simulink model "ClosedLoopPMSM_ASMO_MPC"  (R2023b)
settings: Solver=ode4  StartTime=0.0  StopTime=3  FixedStep=1e-6  RelTol=1e-4
InitFcn:
  | Vdc=24;
  | Rs=0.05734;
  | Ld=1.8166e-05;
  | Lq=1.8166e-05;
  | Ls=1.8166e-05;
  | pm=0.0185;
  | P=14;
  | B=1e-4;
  | J=2.94e-5;
  | Tpwm=30e-6;
  | 
  | fc=20;
  | mag_vel=100;
undefined symbols (not defined in the file): DiscIntNeverNeededParam
libraries: simulink x3, spsThreePhaseVIMeasurementLib x2, spsDCVoltageSourceLib x2, slpidlib x2, spsThreeLevelBridgeLib x1, spsUniversalBridgeLib x1, spsPermanentMagnetSynchronousMachineLib x1, sps_lib x1
(part 1 of 2)
settings Model: Creator=Admin  LastModifiedBy=Admin
settings SolverCC: AlgebraicLoopSolver=TrustRegion
settings DataIOCC: ReturnWorkspaceOutputs=off
settings OptimizationCC: LifeSpan=inf
settings DebuggingCC: UnconnectedInputMsg=warning  UnconnectedOutputMsg=warning  UnconnectedLineMsg=warning  SFUnexpectedBacktrackingDiag=warning  SFNoUnconditionalDefaultTransitionDiag=warning  ArithmeticOperatorsInVariantConditions=warning
settings ModelReferenceCC: EnableRefExpFcnMdlSchedulingChecks=on
settings SFSimCC: SimUseLocalCustomCode=off  CustomCodeUndefinedFunction=UseInterfaceOnly
settings RTWCC: RTWUseLocalCustomCode=off
settings CodeAppCC: StateflowObjectComments=on
settings GRTTargetCC: TargetLangStandard=C89/C90 (ANSI)
settings ConfigComp: CovMetricSettings=dw  CovSaveCumulativeToWorkspaceVar=on  CovSaveSingleToWorkspaceVar=on  CovExternalEMLEnable=off
settings SimscapeCC: SimscapeNormalizeSystem=off

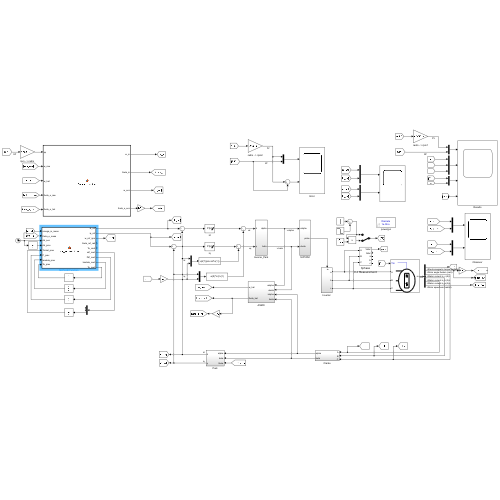
[thumbnail: Simulink's stored preview of the top-level diagram]
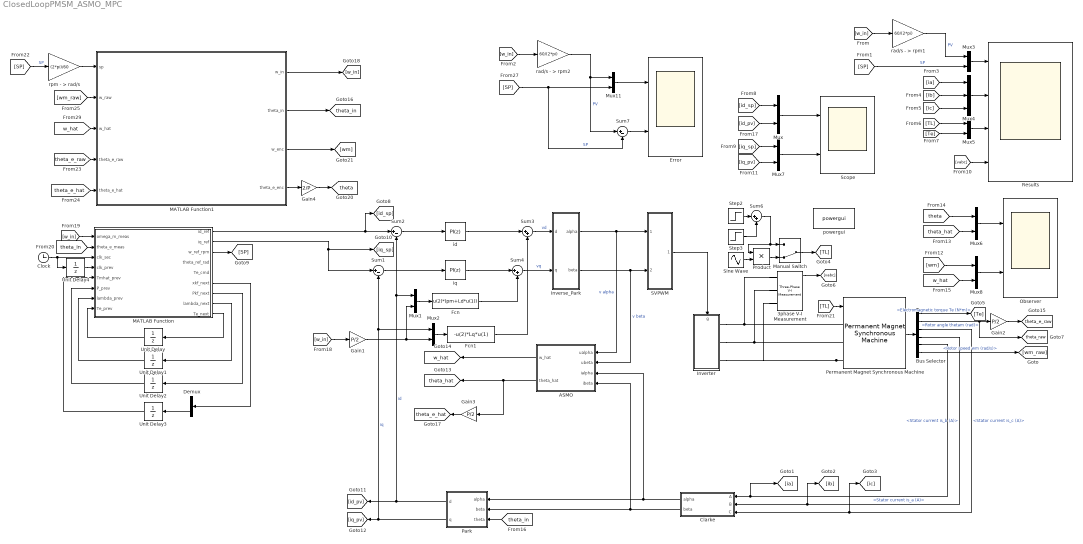
== system ClosedLoopPMSM_ASMO_MPC ==
  3phase V-I Measurement : spsThreePhaseVIMeasurementLib/Three-Phase V-I Measurement  VoltageMeasurement=phase-to-phase  SetLabelV=off  LabelV=Vabc  Vpu=off  VpuLL=off  CurrentMeasurement=yes  SetLabelI=off  LabelI=Iabc  Ipu=off  Pbase=100e6  Vbase=500e3  OutputType=Complex  PhasorSimulation=off  PSBequivalent=0
  ASMO : Subsystem
  Bus Selector : BusSelector  OutputSignals=Electromagnetic torque Te (N*m),Rotor angle thetam (rad),Stator current is_c (A),Stator current is_b (A),Stator current is_a (A),Rotor speed wm (rad/s)
  Clarke : Subsystem
  Clock : Clock
      settings: Decimation=33
  Demux : Demux  Outputs=3
  Error : Scope  NumInputPorts=2
  Fcn : Fcn  Expr=u(2)*(pm+Ld*u(1))
  Fcn1 : Fcn  Expr=-u(2)*Lq*u(1)
  Gain1 : Gain  Gain=P/2
  Gain2 : Gain  Gain=P/2
  Gain3 : Gain  Gain=P/2
  Gain4 : Gain  Gain=2/P
  Inverse_Park : Subsystem
  Inverter : Subsystem
      settings: PortSchema="{\"entries\":[{\"content\":{\"sides\":[{\"content\":{},\"type\":\"ConnectorPlacement.EquallySpacedRectSide\",\"uuid\":\"187c6bc1-a8de-4289-8015-4317398378bc\"},{\"content\":{\"connectorIds\":[\"RConn1\",\"RConn2\",\"RConn3\"],\"side\":\"RIGHT\"},\"type\":\"ConnectorPlacement.EquallySpacedRectSide\",\"uuid\":\"9f177a2c-a1b4-485f-9b91-a35efcc62074\"},{\"content\":{\"connectorIds\":[\"In1\"],\"side\":\"TOP\"},\"type\":\"ConnectorPlacement.EquallySpacedRectSide\",\"uuid\":\"7cd38b0a-0afe-4879-8b43-8c0c1c17e55c\"}]},\"type\":\"ConnectorPlacement.EquallySpacedConnector\",\"uuid\":\"53672e9b-5b63-4df3-a21b-cd886d268e09\"}],\"packageUris\":[\"http://schema.mathworks.com/mf0/Connector/R2020b\"],\"version\":\"1.0\"}"
  MATLAB Function : MATLAB Function  TreatAsAtomicUnit=on
  MATLAB Function1 : MATLAB Function  TreatAsAtomicUnit=on
  Manual Switch : ManualSwitch  CurrentSetting=0
  Mux{,1..3,5..8,11} (9 alike) : Mux  Inputs=2
  Mux4 : Mux  Inputs=3
  Observer : Scope  NumInputPorts=2
  Park : Subsystem
  Permanent Magnet Synchronous Machine : spsPermanentMagnetSynchronousMachineLib/Permanent Magnet Synchronous Machine  NbPhases=3  FluxDistribution=Sinusoidal  RotorType=Salient-pole  MechanicalLoad=Torque Tm  PresetModel=No  ShowDetailedParameters=on  MeasurementBus=off  Resistance=Rs  Inductance=8.5e-3  dqInductances=[Ld,Lq]  La=0.000395  MachineConstant=Flux linkage established by magnets (V.s)  Flux=pm  VoltageCst=23.4887  TorqueCst=0.19425  Flat=120  Mechanical=[J B P/2]  PolePairs=4  InitialConditions=[0,0, 0,0]  InitialConditions5ph=[0 0 0 0 0 0]  RefAngle=Aligned with phase A axis (original Park)  IterativeDiscreteModel=Trapezoidal non iterative  TsBlock=-1  TsPowergui=0
  Product : Product
  Results : Scope  NumInputPorts=4
  SVPWM : Subsystem
  Scope : Scope  NumInputPorts=2
  Sine Wave : Sin  Frequency=62.83  SampleTime=0
  Step2 : Step  Time=0.1  After=0.1  SampleTime=0
  Step3 : Step  Time=0.15  After=-0.1  SampleTime=0
  Sum1 : Sum  Inputs=|+-
  Sum2 : Sum  Inputs=|+-
  Sum3 : Sum  Inputs=|++
  Sum4 : Sum  Inputs=|++
  Sum6 : Sum  Inputs=|++
  Sum7 : Sum  Inputs=|+-
  Unit Delay : UnitDelay  SampleTime=30e-6  HasFrameUpgradeWarning=on
  Unit Delay1 : UnitDelay  InitialCondition=zeros(16,1)  SampleTime=30e-6  HasFrameUpgradeWarning=on
  Unit Delay2 : UnitDelay  InitialCondition=reshape([1 0 0; 0 1 0; 0 0 1], 9, 1)  SampleTime=30e-6  HasFrameUpgradeWarning=on
  Unit Delay3 : UnitDelay  SampleTime=30e-6  HasFrameUpgradeWarning=on
  Unit Delay4 : UnitDelay  SampleTime=30e-6  HasFrameUpgradeWarning=on
  id : slpidlib/PID Controller  Controller=PI  Form=Parallel  TimeDomain=Discrete-time  UseExternalTs=off  SampleTime=-1  IntegratorMethod=Forward Euler  FilterMethod=Forward Euler  ControllerParametersSource=internal  P=0.02283e4  I=72.06e1  UseKiTs=off  D=0  N=100  UseFilter=on  TunerSelectOption=Transfer Function Based (PID Tuner App)  InitialConditionSource=internal  InitialConditionForIntegrator=0  InitialConditionForFilter=0  DifferentiatorICPrevScaledInput=0  ExternalReset=none  TrackingMode=off  Kt=1  LimitOutput=on  SatLimitsSource=internal  UpperSaturationLimit=30  LowerSaturationLimit=-30  LinearizeAsGain=off  AntiWindupMode=clamping  Kb=1  LimitIntegrator=off  UpperIntegratorSaturationLimit=inf  LowerIntegratorSaturationLimit=-inf  POutMin=[]  POutMax=[]  IOutMin=[]  IOutMax=[]  DOutMin=[]  DOutMax=[]  NOutMin=[]  NOutMax=[]  SumOutMin=[]  SumOutMax=[]  SaturationOutMin=[]  SaturationOutMax=[]  PParamMin=[]  PParamMax=[]  IParamMin=[]  IParamMax=[]  DParamMin=[]  DParamMax=[]  NParamMin=[]  NParamMax=[]  KbParamMin=[]  KbParamMax=[]  KtParamMin=[]  KtParamMax=[]  KbOutMin=[]  KbOutMax=[]  KtOutMin=[]  KtOutMax=[]  IntegratorOutMin=[]  IntegratorOutMax=[]  FilterOutMin=[]  FilterOutMax=[]  SumI1OutMin=[]  SumI1OutMax=[]  SumI2OutMin=[]  SumI2OutMax=[]  SumI3OutMin=[]  SumI3OutMax=[]  SumI4OutMin=[]  SumI4OutMax=[]  SumDOutMin=[]  SumDOutMax=[]  DifferentiatorOutMin=[]  DifferentiatorOutMax=[]  FilterDiffOutCoefMin=[]  FilterDiffOutCoefMax=[]  ReciprocalOutMin=[]  ReciprocalOutMax=[]  SumDenOutMin=[]  SumDenOutMax=[]  SumNumOutMin=[]  SumNumOutMax=[]  DivideOutMin=[]  DivideOutMax=[]  UdiffTsProdOutMin=[]  UdiffTsProdOutMax=[]  NTsProdOutMin=[]  NTsProdOutMax=[]  UintegralTsProdOutMin=[]  UintegralTsProdOutMax=[]  UngainTsProdOutMin=[]  UngainTsProdOutMax=[]  ClampingZeroOutDataTypeStr=Inherit: Inherit via back propagation  ClampingZeroOutMin=[]  ClampingZeroOutMax=[]  FilterDenConstantOutDataTypeStr=Inherit: Inherit via back propagation  FilterDenConstantOutMin=[]  FilterDenConstantOutMax=[]  PCopyOutDataTypeStr=Inherit: Inherit via back propagation  PCopyOutMin=[]  PCopyOutMax=[]  NCopyOutDataTypeStr=Inherit: Inherit via back propagation  NCopyOutMin=[]  NCopyOutMax=[]  IntegratorContinuousStateAttributes=''  IntegratorStateMustResolveToSignalObject=off  IntegratorRTWStateStorageClass=Auto  FilterContinuousStateAttributes=''  FilterStateMustResolveToSignalObject=off  FilterRTWStateStorageClass=Auto  ParallelPVariant=InternalParameters  IdealPVariant=Disabled  IVariant=InternalParameters  DVariant=Disabled  IntegratorVariant=Discrete  SatVariant=Enabled  AWVariant=DiscClampingParallel  PCopyVariant=Disabled  TRVariant=Disabled  FdbkBlocksVariant=Forward  IdealPFdbkVariant=Disabled  SatFdbkVariant=Disabled  DerivativeFilterVariant=Disabled  NVariant=Disabled  NCopyVariant=Disabled_SignalSpec  FilterICVariant=Disabled  IntegratorICVariant=InternalICs  ExternalResetVariant=Disabled  TRSumVariant=Passthrough  SumFdbkVariant=Disabled  SumVariant=Sum_PI  TsampFilterVariant=InternalTs  TsampNgainVariant=Passthrough  TsampIntegralVariant=Disabled_SignalSpec  ExternalSaturationOutDataTypeStr=Inherit: Same as second input
  iq : slpidlib/PID Controller  Controller=PI  Form=Parallel  TimeDomain=Discrete-time  UseExternalTs=off  SampleTime=-1  IntegratorMethod=Forward Euler  FilterMethod=Forward Euler  ControllerParametersSource=internal  P=0.02283e4  I=72.06e1  UseKiTs=off  D=0  N=100  UseFilter=on  TunerSelectOption=Transfer Function Based (PID Tuner App)  InitialConditionSource=internal  InitialConditionForIntegrator=0  InitialConditionForFilter=0  DifferentiatorICPrevScaledInput=0  ExternalReset=none  TrackingMode=off  Kt=1  LimitOutput=on  SatLimitsSource=internal  UpperSaturationLimit=30  LowerSaturationLimit=-30  LinearizeAsGain=off  AntiWindupMode=clamping  Kb=1  LimitIntegrator=off  UpperIntegratorSaturationLimit=inf  LowerIntegratorSaturationLimit=-inf  POutMin=[]  POutMax=[]  IOutMin=[]  IOutMax=[]  DOutMin=[]  DOutMax=[]  NOutMin=[]  NOutMax=[]  SumOutMin=[]  SumOutMax=[]  SaturationOutMin=[]  SaturationOutMax=[]  PParamMin=[]  PParamMax=[]  IParamMin=[]  IParamMax=[]  DParamMin=[]  DParamMax=[]  NParamMin=[]  NParamMax=[]  KbParamMin=[]  KbParamMax=[]  KtParamMin=[]  KtParamMax=[]  KbOutMin=[]  KbOutMax=[]  KtOutMin=[]  KtOutMax=[]  IntegratorOutMin=[]  IntegratorOutMax=[]  FilterOutMin=[]  FilterOutMax=[]  SumI1OutMin=[]  SumI1OutMax=[]  SumI2OutMin=[]  SumI2OutMax=[]  SumI3OutMin=[]  SumI3OutMax=[]  SumI4OutMin=[]  SumI4OutMax=[]  SumDOutMin=[]  SumDOutMax=[]  DifferentiatorOutMin=[]  DifferentiatorOutMax=[]  FilterDiffOutCoefMin=[]  FilterDiffOutCoefMax=[]  ReciprocalOutMin=[]  ReciprocalOutMax=[]  SumDenOutMin=[]  SumDenOutMax=[]  SumNumOutMin=[]  SumNumOutMax=[]  DivideOutMin=[]  DivideOutMax=[]  UdiffTsProdOutMin=[]  UdiffTsProdOutMax=[]  NTsProdOutMin=[]  NTsProdOutMax=[]  UintegralTsProdOutMin=[]  UintegralTsProdOutMax=[]  UngainTsProdOutMin=[]  UngainTsProdOutMax=[]  ClampingZeroOutDataTypeStr=Inherit: Inherit via back propagation  ClampingZeroOutMin=[]  ClampingZeroOutMax=[]  FilterDenConstantOutDataTypeStr=Inherit: Inherit via back propagation  FilterDenConstantOutMin=[]  FilterDenConstantOutMax=[]  PCopyOutDataTypeStr=Inherit: Inherit via back propagation  PCopyOutMin=[]  PCopyOutMax=[]  NCopyOutDataTypeStr=Inherit: Inherit via back propagation  NCopyOutMin=[]  NCopyOutMax=[]  IntegratorContinuousStateAttributes=''  IntegratorStateMustResolveToSignalObject=off  IntegratorRTWStateStorageClass=Auto  FilterContinuousStateAttributes=''  FilterStateMustResolveToSignalObject=off  FilterRTWStateStorageClass=Auto  ParallelPVariant=InternalParameters  IdealPVariant=Disabled  IVariant=InternalParameters  DVariant=Disabled  IntegratorVariant=Discrete  SatVariant=Enabled  AWVariant=DiscClampingParallel  PCopyVariant=Disabled  TRVariant=Disabled  FdbkBlocksVariant=Forward  IdealPFdbkVariant=Disabled  SatFdbkVariant=Disabled  DerivativeFilterVariant=Disabled  NVariant=Disabled  NCopyVariant=Disabled_SignalSpec  FilterICVariant=Disabled  IntegratorICVariant=InternalICs  ExternalResetVariant=Disabled  TRSumVariant=Passthrough  SumFdbkVariant=Disabled  SumVariant=Sum_PI  TsampFilterVariant=InternalTs  TsampNgainVariant=Passthrough  TsampIntegralVariant=Disabled_SignalSpec  ExternalSaturationOutDataTypeStr=Inherit: Same as second input
  powergui : sps_lib/powergui  Priority=1  SimulationMode=Discrete  SampleTime=1e-6  frequency=60  Iterations=50  frequencyindice=0  Pbase=100e6  ErrMax=1e-4  UnitsV=kV  UnitsW=MW  buscounter=0  FunctionMessages=off  echomessages=off  EnableUseOfTLC=off  CurrentSourceSwitches=on  DisableSnubberDevices=off  DisableRonSwitches=off  DisableVfSwitches=off  DisplayEquations=off  AutomaticDiscreteSolvers=off  SolverType=Tustin/Backward Euler (TBE)  Interpol=off  ExternalGateDelay=off  methode=off  Ts=100  x0status=blocks  SPID=on  SwTol=0  HookPort=off  NonlinearTolerance=1e-4  nMaxIteration=100  ContinueOnMaxIteration=off  RestoreLinks=warning  ResistiveCurrentMeasurement=off  Frange=[0:2:500]  Ylog=off  Xlog=on  ShowGrid=off  save=off  variable=ZData  structure=0  ZoomFFT=off  StartTime=0.0  cycles=1  DisplayStyle=1  fundamental=60  FreqAxis=off  MaxFrequency=1000  frequencyindicesteady=1  RmsSteady=1  display=off
  rad/s - > rpm1 : Gain  Gain=60/(2*pi)
  rad/s - > rpm2 : Gain  Gain=60/(2*pi)
  "rpm - > rad/s " : Gain  Gain=(2*pi)/60
  tag scope: theta=global, theta_e_hat=global, theta_e_raw=global, theta_hat=global, theta_in=global, theta_raw=global, w_hat=global
  wires:
  Park/1(d) -> Sum2/2, Mux1/1, [id_pv]  "id"
  Park/2(q) -> Sum1/2, Mux2/1, [iq_pv]  "iq"
  Mux1/1 -> Fcn/1
  Mux2/1 -> Fcn1/1
  Permanent Magnet Synchronous Machine/1 -> Bus Selector/1
  Bus Selector/3 -> Clarke/3(C), [ic]  "<Stator current is_c (A)>"
  Bus Selector/4 -> Clarke/2(B), [ib]  "<Stator current is_b (A)>"
  Bus Selector/5 -> Clarke/1(A), [ia]  "<Stator current is_a (A)>"
  Gain1/1 -> Mux1/2, Mux2/2
  3phase V-I Measurement/1 -> [vabc]
  Sum3/1 -> Inverse_Park/1(d)  "vd"
  Sum4/1 -> Inverse_Park/2(q)  "vq"
  SVPWM/1(pulse) -> Inverter/1(g)
  Inverse_Park/1(alpha) -> ASMO/1(ualpha), SVPWM/1(valpha)  "v alpha"
  Inverse_Park/2(beta) -> ASMO/2(ubeta), SVPWM/2(vbeta)  "v beta"
  Gain2/1 -> [theta_e_raw]
  Bus Selector/6 -> [wm_raw]  "<Rotor speed wm (rad/s)>"
  Sum2/1 -> id/1
  Sum1/1 -> iq/1
  Fcn/1 -> Sum4/2
  Fcn1/1 -> Sum3/2
  Gain3/1 -> [theta_e_hat]
  ASMO/2(theta_hat) -> [theta_hat], Gain3/1
  Clarke/2(beta) -> ASMO/4(ibeta), Park/2(beta)
  Clarke/1(alpha) -> ASMO/3(ialpha), Park/1(alpha)
  ASMO/1(w_hat) -> [w_hat]
  id/1 -> Sum3/1
  iq/1 -> Sum4/1
  Bus Selector/2 -> [theta_raw], Gain2/1  "<Rotor angle thetam (rad)>"
  [TL] -> Permanent Magnet Synchronous Machine/1
  Clock/1 -> MATLAB Function/3(clk_sec), Unit Delay4/1
  MATLAB Function/9(Te_next) -> Unit Delay/1
  Unit Delay/1 -> MATLAB Function/8(Te_prev)
  MATLAB Function/8(lambda_next) -> Unit Delay1/1
  Unit Delay1/1 -> MATLAB Function/7(lambda_prev)
  MATLAB Function/7(Pkf_next) -> Unit Delay2/1
  Unit Delay2/1 -> MATLAB Function/6(P_prev)
  Unit Delay3/1 -> MATLAB Function/5(Tmhat_prev)
  Unit Delay4/1 -> MATLAB Function/4(clk_prev)
  MATLAB Function/1(id_ref) -> [id_sp], Sum2/1
  MATLAB Function/3(w_ref_rpm) -> [SP]
  MATLAB Function/6(xkf_next) -> Demux/1
  Demux/3 -> Unit Delay3/1
  Bus Selector/1 -> [Te]  "<Electromagnetic torque Te (N*m)>"
  MATLAB Function1/4(theta_e_enc) -> Gain4/1
  MATLAB Function1/3(w_enc) -> [wm]
  [w_hat] -> MATLAB Function1/3(w_hat)
  MATLAB Function1/1(w_in) -> [w_in]
  MATLAB Function1/2(theta_in) -> [theta_in]
  [theta_e_hat] -> MATLAB Function1/5(theta_e_hat)
  "rpm - > rad/s "/1 -> MATLAB Function1/1(sp)
  Gain4/1 -> [theta]
  [theta_e_raw] -> MATLAB Function1/4(theta_e_raw)
  [SP] -> "rpm - > rad/s "/1  "SP"
  [wm_raw] -> MATLAB Function1/2(w_raw)
  [w_in] -> Gain1/1
  [w_in] -> MATLAB Function/1(omega_m_meas)
  [theta_in] -> Park/3(theta)
  rad/s - > rpm2/1 -> Sum7/1, Mux11/1  "PV"
  [SP] -> Mux3/2  "SP"
  [iq_pv] -> Mux7/2
  [w_in] -> rad/s - > rpm2/1
  [ia] -> Mux4/1
  [ic] -> Mux4/3
  [SP] -> Sum7/2, Mux11/2  "SP"
  Mux11/1 -> Error/1
  Sum7/1 -> Error/2
  Mux7/1 -> Scope/2
  Mux5/1 -> Results/3
  [iq_sp] -> Mux7/1
  [id_sp] -> Mux/1
  rad/s - > rpm1/1 -> Mux3/1  "PV"
  [TL] -> Mux5/1
  [vabc] -> Results/4
  [ib] -> Mux4/2
  Mux/1 -> Scope/1
  [id_pv] -> Mux/2
  Mux3/1 -> Results/1
  [w_in] -> rad/s - > rpm1/1
  [Te] -> Mux5/2
  Mux4/1 -> Results/2
  [wm] -> Mux8/1
  Mux6/1 -> Observer/1
  [w_hat] -> Mux8/2
  Mux8/1 -> Observer/2
  [theta] -> Mux6/1
  [theta_hat] -> Mux6/2
  MATLAB Function/2(iq_ref) -> Sum1/1, [iq_sp]
  [theta_in] -> MATLAB Function/2(theta_e_meas)
  Step2/1 -> Sum6/1
  Step3/1 -> Sum6/2
  Sum6/1 -> Product/1, Manual Switch/1
  Product/1 -> Manual Switch/2
  Sine Wave/1 -> Product/2
  Manual Switch/1 -> [TL]
  connections:
  3phase V-I Measurement/LConn1 -- Inverter/RConn1 -- Permanent Magnet Synchronous Machine/LConn1
  3phase V-I Measurement/LConn2 -- Inverter/RConn2 -- Permanent Magnet Synchronous Machine/LConn2
  Permanent Magnet Synchronous Machine/LConn3 -- Inverter/RConn3 -- 3phase V-I Measurement/LConn3

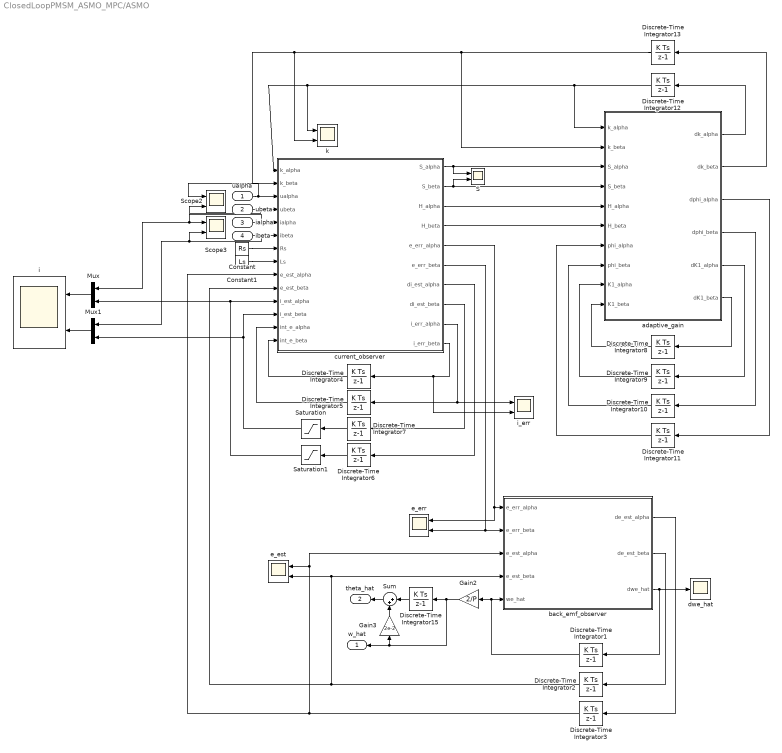
== system ClosedLoopPMSM_ASMO_MPC/ASMO ==
  ualpha : Inport
  ubeta : Inport  Port=2
  ialpha : Inport  Port=3
  ibeta : Inport  Port=4
  Constant : Constant  Value=Rs
  Constant1 : Constant  Value=Ls
  Discrete-Time Integrator1 : DiscreteIntegrator  gainval=2.5e2*3  SampleTime=-1  ICPrevOutput=DiscIntNeverNeededParam  ICPrevScaledInput=DiscIntNeverNeededParam
  Discrete-Time Integrator{2..5,8..11} (8 alike) : DiscreteIntegrator  SampleTime=-1  ICPrevOutput=DiscIntNeverNeededParam  ICPrevScaledInput=DiscIntNeverNeededParam
  Discrete-Time Integrator12 : DiscreteIntegrator  InitialCondition=50  SampleTime=-1  ICPrevOutput=DiscIntNeverNeededParam  ICPrevScaledInput=DiscIntNeverNeededParam
  Discrete-Time Integrator13 : DiscreteIntegrator  InitialCondition=50  SampleTime=-1  ICPrevOutput=DiscIntNeverNeededParam  ICPrevScaledInput=DiscIntNeverNeededParam
  Discrete-Time Integrator15 : DiscreteIntegrator  gainval=1  SampleTime=-1  ICPrevOutput=DiscIntNeverNeededParam  ICPrevScaledInput=DiscIntNeverNeededParam
  Discrete-Time Integrator6 : DiscreteIntegrator  gainval=1.0e-2*5  SampleTime=-1  ICPrevOutput=DiscIntNeverNeededParam  ICPrevScaledInput=DiscIntNeverNeededParam
  Discrete-Time Integrator7 : DiscreteIntegrator  gainval=1.0e-2*5  SampleTime=-1  ICPrevOutput=DiscIntNeverNeededParam  ICPrevScaledInput=DiscIntNeverNeededParam
  Gain2 : Gain  Gain=2/P
  Gain3 : Gain  Gain=2e-2
  Mux : Mux  Inputs=2
  Mux1 : Mux  Inputs=2
  S : Scope  NumInputPorts=2
  Saturation : Saturate  UpperLimit=2  LowerLimit=-2
  Saturation1 : Saturate  UpperLimit=2  LowerLimit=-2
  Scope2 : Scope  NumInputPorts=2
  Scope3 : Scope  NumInputPorts=2
  Sum : Sum  Inputs=|++
  adaptive_gain : MATLAB Function  TreatAsAtomicUnit=on
  back_emf_observer : MATLAB Function  TreatAsAtomicUnit=on
  current_observer : MATLAB Function  TreatAsAtomicUnit=on
  dwe_hat : Scope
  e_err : Scope  NumInputPorts=2
  e_est : Scope  NumInputPorts=2
  i : Scope  NumInputPorts=2
  i_err : Scope  NumInputPorts=2
  k : Scope  NumInputPorts=2
  w_hat : Outport
  theta_hat : Outport  Port=2
  wires:
  ualpha/1 -> Scope2/1, current_observer/3(ualpha)
  ubeta/1 -> current_observer/4(ubeta), Scope2/2
  ialpha/1 -> Mux/1, Scope3/1, current_observer/5(ialpha)
  ibeta/1 -> Scope3/2, Mux1/1, current_observer/6(ibeta)
  Constant/1 -> current_observer/7(Rs)
  Constant1/1 -> current_observer/8(Ls)
  current_observer/7(di_est_alpha) -> Discrete-Time Integrator6/1
  current_observer/8(di_est_beta) -> Discrete-Time Integrator7/1
  current_observer/1(S_alpha) -> adaptive_gain/3(S_alpha), S/1
  current_observer/2(S_beta) -> S/2, adaptive_gain/4(S_beta)
  current_observer/3(H_alpha) -> adaptive_gain/5(H_alpha)
  current_observer/4(H_beta) -> adaptive_gain/6(H_beta)
  adaptive_gain/3(dphi_alpha) -> Discrete-Time Integrator11/1
  adaptive_gain/4(dphi_beta) -> Discrete-Time Integrator10/1
  adaptive_gain/5(dK1_alpha) -> Discrete-Time Integrator9/1
  adaptive_gain/6(dK1_beta) -> Discrete-Time Integrator8/1
  adaptive_gain/1(dk_alpha) -> Discrete-Time Integrator12/1
  adaptive_gain/2(dk_beta) -> Discrete-Time Integrator13/1
  back_emf_observer/1(de_est_alpha) -> Discrete-Time Integrator3/1
  back_emf_observer/2(de_est_beta) -> Discrete-Time Integrator2/1
  Discrete-Time Integrator4/1 -> current_observer/14(int_e_beta)
  Discrete-Time Integrator5/1 -> current_observer/13(int_e_alpha)
  Discrete-Time Integrator7/1 -> Saturation/1
  Discrete-Time Integrator6/1 -> Saturation1/1
  Discrete-Time Integrator8/1 -> adaptive_gain/10(K1_beta)
  Discrete-Time Integrator9/1 -> adaptive_gain/9(K1_alpha)
  Discrete-Time Integrator10/1 -> adaptive_gain/8(phi_beta)
  Discrete-Time Integrator11/1 -> adaptive_gain/7(phi_alpha)
  Discrete-Time Integrator13/1 -> adaptive_gain/2(k_beta), k/2, current_observer/2(k_beta)
  Discrete-Time Integrator12/1 -> adaptive_gain/1(k_alpha), k/1, current_observer/1(k_alpha)
  current_observer/9(i_err_alpha) -> Discrete-Time Integrator5/1, i_err/1
  current_observer/10(i_err_beta) -> Discrete-Time Integrator4/1, i_err/2
  current_observer/5(e_err_alpha) -> e_err/1, back_emf_observer/1(e_err_alpha)
  current_observer/6(e_err_beta) -> e_err/2, back_emf_observer/2(e_err_beta)
  back_emf_observer/3(dwe_hat) -> Discrete-Time Integrator1/1, dwe_hat/1
  Discrete-Time Integrator2/1 -> current_observer/10(e_est_beta), e_est/2, back_emf_observer/4(e_est_beta)
  Discrete-Time Integrator3/1 -> current_observer/9(e_est_alpha), e_est/1, back_emf_observer/3(e_est_alpha)
  Discrete-Time Integrator15/1 -> Sum/1
  Sum/1 -> theta_hat/1
  Gain2/1 -> Discrete-Time Integrator15/1, Gain3/1, w_hat/1
  Gain3/1 -> Sum/2
  Mux/1 -> i/1
  Mux1/1 -> i/2
  Discrete-Time Integrator1/1 -> back_emf_observer/5(we_hat), Gain2/1
  Saturation/1 -> current_observer/12(i_est_beta), Mux1/2
  Saturation1/1 -> current_observer/11(i_est_alpha), Mux/2

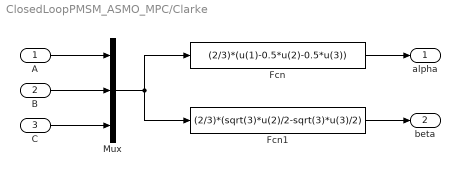
== system ClosedLoopPMSM_ASMO_MPC/Clarke ==
  A : Inport
  B : Inport  Port=2
  C : Inport  Port=3
  Fcn : Fcn  Expr=(2/3)*(u(1)-0.5*u(2)-0.5*u(3))
  Fcn1 : Fcn  Expr=(2/3)*(sqrt(3)*u(2)/2-sqrt(3)*u(3)/2)
  Mux : Mux  Inputs=3
  alpha : Outport
  beta : Outport  Port=2
  wires:
  B/1 -> Mux/2
  A/1 -> Mux/1
  C/1 -> Mux/3
  Mux/1 -> Fcn1/1, Fcn/1
  Fcn/1 -> alpha/1
  Fcn1/1 -> beta/1

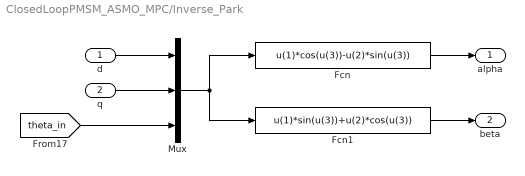
== system ClosedLoopPMSM_ASMO_MPC/Inverse_Park ==
  d : Inport
  q : Inport  Port=2
  Fcn : Fcn  Expr=u(1)*cos(u(3))-u(2)*sin(u(3))
  Fcn1 : Fcn  Expr=u(1)*sin(u(3))+u(2)*cos(u(3))
  Mux : Mux  Inputs=3
  alpha : Outport
  beta : Outport  Port=2
  wires:
  Fcn1/1 -> beta/1
  d/1 -> Mux/1
  q/1 -> Mux/2
  Mux/1 -> Fcn1/1, Fcn/1
  Fcn/1 -> alpha/1
  [theta_in] -> Mux/3

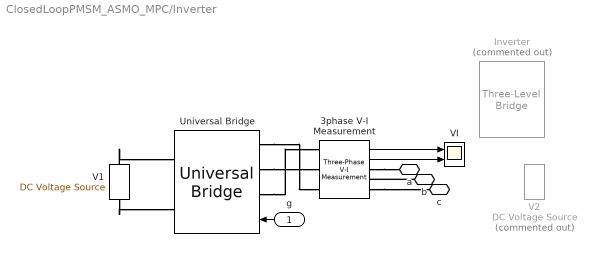
== system ClosedLoopPMSM_ASMO_MPC/Inverter ==
  g : Inport
  3phase V-I Measurement : spsThreePhaseVIMeasurementLib/Three-Phase V-I Measurement  VoltageMeasurement=phase-to-phase  SetLabelV=off  LabelV=Vabc  Vpu=off  VpuLL=off  CurrentMeasurement=yes  SetLabelI=off  LabelI=Iabc  Ipu=off  Pbase=100e6  Vbase=500e3  OutputType=Complex  PhasorSimulation=off  PSBequivalent=0
  Inverter : spsThreeLevelBridgeLib/Three-Level Bridge  Commented=on  Arms=3  SnubberResistance=1e5  SbubberCapacitance=1e-8  Device=IGBT / Diodes  Ron=0.2e-7  ForwardVoltages=[0.1 0.1]  Measurements=All voltages and currents
      settings: AttributesFormatString=\n
  Universal Bridge : spsUniversalBridgeLib/Universal Bridge  Arms=3  SnubberResistance=1e5  SnubberCapacitance=1e-8  Device=MOSFET / Diodes  Ron=0.2e-7  Lon=0  ForwardVoltages="[  0  0  ]"  ForwardVoltage=0  GTOparameters=[ 10e-6 , 20e-6 ]  IGBTparameters=[ 1e-6 , 2e-6 ]  Measurements=All voltages and currents  Measurements_2=None  converterType=Rectifier
  V1 : spsDCVoltageSourceLib/DC Voltage Source  Amplitude=Vdc  Measurements=None
  V2 : spsDCVoltageSourceLib/DC Voltage Source  Commented=on  Amplitude=Vdc/2  Measurements=None
  VI : Scope  NumInputPorts=2
  a : PMIOPort  Side=Right
  b : PMIOPort  Port=2  Side=Right
  c : PMIOPort  Port=3  Side=Right
  wires:
  3phase V-I Measurement/2 -> VI/2
  3phase V-I Measurement/1 -> VI/1
  g/1 -> Universal Bridge/1
  connections:
  3phase V-I Measurement/RConn3 -- c/RConn1
  b/RConn1 -- 3phase V-I Measurement/RConn2
  3phase V-I Measurement/RConn1 -- a/RConn1
  Universal Bridge/LConn3 -- 3phase V-I Measurement/LConn3
  Universal Bridge/LConn2 -- 3phase V-I Measurement/LConn2
  Universal Bridge/LConn1 -- 3phase V-I Measurement/LConn1
  V1/RConn1 -- Universal Bridge/RConn1
  V1/LConn1 -- Universal Bridge/RConn2

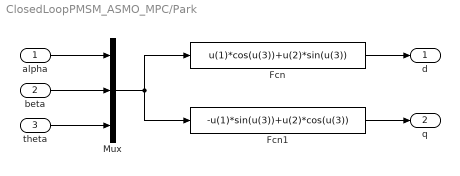
== system ClosedLoopPMSM_ASMO_MPC/Park ==
  alpha : Inport
  beta : Inport  Port=2
  theta : Inport  Port=3
  Fcn : Fcn  Expr=u(1)*cos(u(3))+u(2)*sin(u(3))
  Fcn1 : Fcn  Expr=-u(1)*sin(u(3))+u(2)*cos(u(3))
  Mux : Mux  Inputs=3
  d : Outport
  q : Outport  Port=2
  wires:
  beta/1 -> Mux/2
  alpha/1 -> Mux/1
  Mux/1 -> Fcn1/1, Fcn/1
  Fcn/1 -> d/1
  Fcn1/1 -> q/1
  theta/1 -> Mux/3

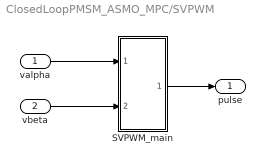
== system ClosedLoopPMSM_ASMO_MPC/SVPWM ==
  valpha : Inport
  vbeta : Inport  Port=2
  SVPWM_main : Subsystem
  pulse : Outport
  wires:
  SVPWM_main/1(pulse) -> pulse/1
  valpha/1 -> SVPWM_main/1(Ualpha)
  vbeta/1 -> SVPWM_main/2(Ubeta)

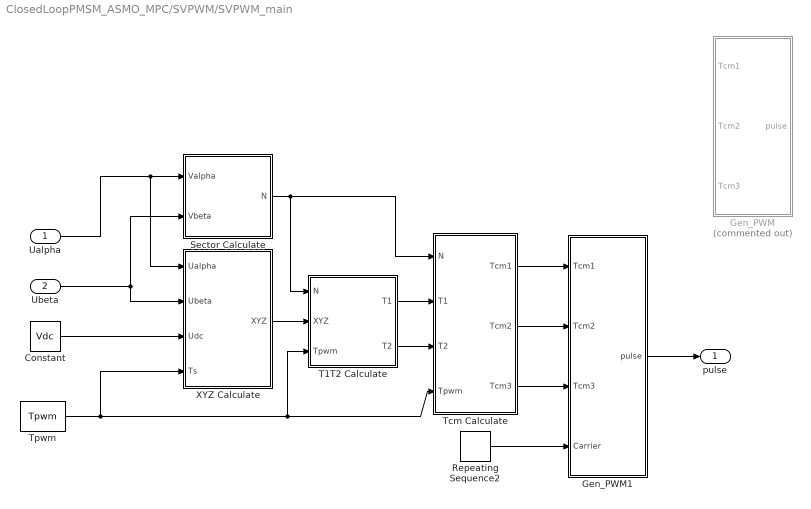
== system ClosedLoopPMSM_ASMO_MPC/SVPWM/SVPWM_main ==
  Ualpha : Inport
  Ubeta : Inport  Port=2
  Constant : Constant  Value=Vdc
  Gen_PWM : Subsystem  Commented=on
  Gen_PWM1 : Subsystem
  Repeating Sequence2 : simulink/Sources/Repeating Sequence  rep_seq_t=[0 Tpwm/2 Tpwm]  rep_seq_y=[0 Tpwm/8 0]
  Sector Calculate : MATLAB Function  TreatAsAtomicUnit=on
  T1T2 Calculate : MATLAB Function  TreatAsAtomicUnit=on
  Tcm Calculate : MATLAB Function  TreatAsAtomicUnit=on
  Tpwm : Constant  Value=Tpwm
  XYZ Calculate : MATLAB Function  TreatAsAtomicUnit=on
  pulse : Outport
  wires:
  Tpwm/1 -> XYZ Calculate/4(Ts), T1T2 Calculate/3(Tpwm), Tcm Calculate/4(Tpwm)
  Sector Calculate/1(N) -> Tcm Calculate/1(N), T1T2 Calculate/1(N)
  Ualpha/1 -> Sector Calculate/1(Valpha), XYZ Calculate/1(Ualpha)
  T1T2 Calculate/1(T1) -> Tcm Calculate/2(T1)
  Ubeta/1 -> Sector Calculate/2(Vbeta), XYZ Calculate/2(Ubeta)
  XYZ Calculate/1(XYZ) -> T1T2 Calculate/2(XYZ)
  Constant/1 -> XYZ Calculate/3(Udc)
  T1T2 Calculate/2(T2) -> Tcm Calculate/3(T2)
  Tcm Calculate/1(Tcm1) -> Gen_PWM1/1(Tcm1)
  Tcm Calculate/2(Tcm2) -> Gen_PWM1/2(Tcm2)
  Tcm Calculate/3(Tcm3) -> Gen_PWM1/3(Tcm3)
  Repeating Sequence2/1 -> Gen_PWM1/4(Carrier)
  Gen_PWM1/1(pulse) -> pulse/1

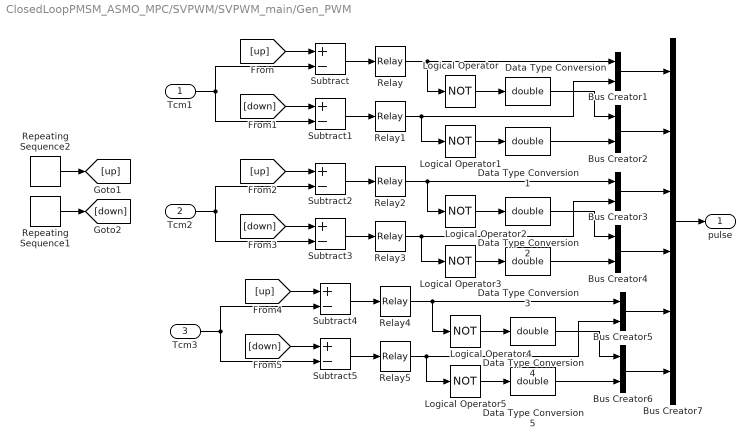
== system ClosedLoopPMSM_ASMO_MPC/SVPWM/SVPWM_main/Gen_PWM ==
  Tcm1 : Inport
  Tcm2 : Inport  Port=2
  Tcm3 : Inport  Port=3
  Bus Creator{1..6} (6 alike) : BusCreator  Inputs=2
  Bus Creator7 : BusCreator  Inputs=6
  Data Type Conversion{,1..5} (6 alike) : DataTypeConversion  OutDataTypeStr=double  SaturateOnIntegerOverflow=off  RndMeth=Floor
  Logical Operator{,1..5} (6 alike) : Logic  Operator=NOT  AllPortsSameDT=off
  Relay{,1..5} (6 alike) : Relay
  Repeating Sequence1 : simulink/Sources/Repeating Sequence  rep_seq_t=[0 Tpwm/2 Tpwm]  rep_seq_y=[Tpwm/4 Tpwm/2 Tpwm/4]
  Repeating Sequence2 : simulink/Sources/Repeating Sequence  rep_seq_t=[0 Tpwm/2 Tpwm]  rep_seq_y=[0 Tpwm/4 0]
  Subtract{,1..5} (6 alike) : Sum  Inputs=+-
  pulse : Outport
  wires:
  Relay1/1 -> Bus Creator1/2, Logical Operator1/1
  Relay/1 -> Bus Creator1/1, Logical Operator/1
  Logical Operator/1 -> Data Type Conversion/1
  Logical Operator1/1 -> Data Type Conversion1/1
  Subtract1/1 -> Relay1/1
  Subtract/1 -> Relay/1
  Bus Creator1/1 -> Bus Creator7/1
  Bus Creator2/1 -> Bus Creator7/2
  Bus Creator7/1 -> pulse/1
  Repeating Sequence2/1 -> [up]
  Tcm1/1 -> Subtract/2, Subtract1/2
  Repeating Sequence1/1 -> [down]
  [up] -> Subtract/1
  [down] -> Subtract1/1
  Data Type Conversion1/1 -> Bus Creator2/2
  Data Type Conversion/1 -> Bus Creator2/1
  Tcm2/1 -> Subtract2/2, Subtract3/2
  Subtract3/1 -> Relay3/1
  Bus Creator3/1 -> Bus Creator7/3
  Bus Creator4/1 -> Bus Creator7/4
  Relay2/1 -> Bus Creator3/1, Logical Operator2/1
  Logical Operator2/1 -> Data Type Conversion2/1
  Relay3/1 -> Bus Creator3/2, Logical Operator3/1
  [up] -> Subtract2/1
  Subtract2/1 -> Relay2/1
  [down] -> Subtract3/1
  Data Type Conversion2/1 -> Bus Creator4/1
  Tcm3/1 -> Subtract4/2, Subtract5/2
  Subtract5/1 -> Relay5/1
  Bus Creator5/1 -> Bus Creator7/5
  Bus Creator6/1 -> Bus Creator7/6
  Relay4/1 -> Bus Creator5/1, Logical Operator4/1
  Logical Operator4/1 -> Data Type Conversion4/1
  Relay5/1 -> Bus Creator5/2, Logical Operator5/1
  [up] -> Subtract4/1
  Subtract4/1 -> Relay4/1
  [down] -> Subtract5/1
  Data Type Conversion4/1 -> Bus Creator6/1
  Data Type Conversion3/1 -> Bus Creator4/2
  Data Type Conversion5/1 -> Bus Creator6/2
  Logical Operator5/1 -> Data Type Conversion5/1
  Logical Operator3/1 -> Data Type Conversion3/1

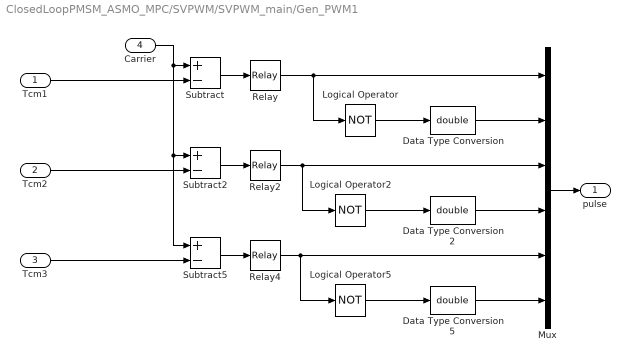
== system ClosedLoopPMSM_ASMO_MPC/SVPWM/SVPWM_main/Gen_PWM1 ==
  Tcm1 : Inport
  Tcm2 : Inport  Port=2
  Tcm3 : Inport  Port=3
  Carrier : Inport  Port=4
  Data Type Conversion : DataTypeConversion  OutDataTypeStr=double  SaturateOnIntegerOverflow=off  RndMeth=Floor
  Data Type Conversion2 : DataTypeConversion  OutDataTypeStr=double  SaturateOnIntegerOverflow=off  RndMeth=Floor
  Data Type Conversion5 : DataTypeConversion  OutDataTypeStr=double  SaturateOnIntegerOverflow=off  RndMeth=Floor
  Logical Operator : Logic  Operator=NOT  AllPortsSameDT=off
  Logical Operator2 : Logic  Operator=NOT  AllPortsSameDT=off
  Logical Operator5 : Logic  Operator=NOT  AllPortsSameDT=off
  Mux : Mux  Inputs=6
  Relay : Relay
  Relay2 : Relay
  Relay4 : Relay
  Subtract : Sum  Inputs=+-
  Subtract2 : Sum  Inputs=+-
  Subtract5 : Sum  Inputs=+-
  pulse : Outport
  wires:
  Relay/1 -> Mux/1, Logical Operator/1
  Logical Operator/1 -> Data Type Conversion/1
  Subtract/1 -> Relay/1
  Mux/1 -> pulse/1
  Tcm2/1 -> Subtract2/2
  Relay2/1 -> Logical Operator2/1, Mux/3
  Logical Operator2/1 -> Data Type Conversion2/1
  Tcm3/1 -> Subtract5/2
  Subtract5/1 -> Relay4/1
  Relay4/1 -> Logical Operator5/1, Mux/5
  Logical Operator5/1 -> Data Type Conversion5/1
  Tcm1/1 -> Subtract/2
  Carrier/1 -> Subtract5/1, Subtract2/1, Subtract/1
  Data Type Conversion5/1 -> Mux/6
  Data Type Conversion2/1 -> Mux/4
  Subtract2/1 -> Relay2/1
  Data Type Conversion/1 -> Mux/2

== matlab function ClosedLoopPMSM_ASMO_MPC/ASMO/back_emf_observer ==
  data: e_err_alpha input; de_est_alpha output; e_err_beta input; e_est_alpha input; e_est_beta input; we_hat input; de_est_beta output; dwe_hat output
function [de_est_alpha, de_est_beta, dwe_hat] = back_emf_observer( ...
    e_err_alpha, e_err_beta, e_est_alpha, e_est_beta, we_hat)

    % --- 1. THAM SO ---
    l_gain = 2e3;  % Tham so l quyet dinh toc do hoi tu 

    % --- 2. UOC LUONG TOC DO ---
    dwe_hat = (e_err_alpha * e_est_beta) - (e_err_beta * e_est_alpha);
    
    % --- 3. CAP NHAT BO QUAN SAT BACK-EMF ---
    % de_est_alpha/dt = -we_hat * e_est_beta - l * tilde_e_alpha 
    % de_est_beta/dt  =  we_hat * e_est_alpha - l * tilde_e_beta 
    
    de_est_alpha = (-we_hat * e_est_beta) - (l_gain * e_err_alpha); 
    de_est_beta  = ( we_hat * e_est_alpha) - (l_gain * e_err_beta);  
    
end

== matlab function ClosedLoopPMSM_ASMO_MPC/MATLAB Function ==
  data: id_ref output; omega_m_meas input; iq_ref output; w_ref_rpm output; theta_ref_rad output; theta_e_meas input; clk_sec input; clk_prev input; Tmhat_prev input; P_prev input; lambda_prev input; Te_prev input; Te_cmd output; xkf_next output; Pkf_next output; lambda_next output; Te_next output
function [id_ref, iq_ref, w_ref_rpm, theta_ref_rad, Te_cmd, xkf_next, Pkf_next, lambda_next, Te_next] = ...
    mpc_kalmannfilter(omega_m_meas, theta_e_meas, clk_sec, clk_prev, ...
                      Tmhat_prev, P_prev, lambda_prev, Te_prev)
% INPUT:
% omega_m_meas [rad/s] - toc do co do duoc
% theta_e_meas [rad]   - goc dien do duoc
% clk_sec [s]          - thoi gian hien tai
% clk_prev [s]         - thoi gian truoc do
% Te_prev [Nm]         - moment dien truoc do
% Tmhat_prev [Nm]      - uoc luong tai truoc do
% P_prev [-]           - ma tran hiep phuong sai KF 
% lambda_prev [-]      - bien doi ngau QP truoc do

% OUTPUT:
% iq_ref [A]           - dong truc q tham chieu
% id_ref [A]           - dong truc d tham chieu
% Te_cmd [Nm]          - moment dua vao vong dong
% xkf_next [-]         - trang thai KF moi (3x1)
% Pkf_next [-]         - ma tran P moi (9x1 reshape)
% lambda_next [-]      - bien doi ngau QP moi
% Te_next [Nm]         - moment sau MPC
% w_ref_rpm [rpm]      - toc do tham chieu
% theta_ref_rad [rad]  - goc tham chieu

% ---------------------------------------------------------
% 0) KHOI TAO NGO RA
% ---------------------------------------------------------
iq_ref        = 0.0;   % [A]
id_ref        = 0.0;   % [A]
Te_cmd        = 0.0;   % [Nm]
xkf_next      = zeros(3,1); 
Pkf_next      = zeros(9,1);
lambda_next   = zeros(16,1); % 2*Nc
Te_next       = 0.0;   % [Nm]
w_ref_rpm     = 0.0;   % [rpm]
theta_ref_rad = 0.0;   % [rad]

%% =======================
% 1) THAM SO
% =======================
Ts        = 30e-6;   % [s]
J         = 2.94e-5; % [kg.m^2]
B         = 1e-4;    % [Nms]
pm        = 0.0185;  % [Wb]
P_poles   = 14;      
p         = P_poles/2;

% MPC
Np        = 25;      % horizon du doan
Nc        = 8;       % horizon dieu khien
Qw        = 300.0;   % trong so toc do
Qth       = 0.5;     % trong so goc
Ru        = 1.8;     % trong so input
Iq_max    = 12.0;    % [A]
Te_max    = 1.5*p*pm*Iq_max; % [Nm]
max_iter  = 200;     % lap toi da QP
tol       = 1e-9;    % dieu kien dung

% KF
q_w  = 0.1;    % nhieu trang thai w
q_th = 1e-9;   % nhieu trang thai theta
q_tm = 0.5;    % nhieu tai
r_w  = 5e-4;   % nhieu do w
r_th = 1e-4;   % nhieu do theta

% Trajectory
mode_traj  = uint8(3); % che do quy dao
MAX_RPM    = 700;
OMEGA_MAX  = MAX_RPM*2*pi/60; % [rad/s]
alpha_max  = 200.0;   % [rad/s^2]
omega_max  = min(100.0, OMEGA_MAX); % [rad/s]
theta_max  = 5.0 * 2 * pi; % [rad]
omega_sin  = 2*pi*2.0; % [rad/s]
wAref      = min(50.0, OMEGA_MAX); % [rad/s]
t1_trap    = omega_max/alpha_max; % [s]
t2_trap    = 0.5; % [s]
t_step     = 1.0; % [s]

%% =======================
% 2) DONG BO CLOCK
% =======================
clk_now_val = clk_sec(1);   % [s]
clk_pre_val = clk_prev(1);  % [s]
new_tick = (clk_now_val > clk_pre_val) || (clk_now_val == 0); % co tick moi

%% ====================================
% 3) KALMAN FILTER
% ====================================
w_m_val  = omega_m_meas(1); % [rad/s]

% doi sang goc co
th_m_val = theta_e_meas(1) / p; % [rad]

Te_p_val = Te_prev(1);     % [Nm]
Tm_p_val = Tmhat_prev(1);  % [Nm]

% ma tran he thong KF
A_kf = [1 - Ts*B/J, 0,        -Ts/J;
        Ts,         1,        0;
        0,          0,        1];

B_kf = [Ts/J; 0; 0];
C_kf = [1 0 0;
        0 1 0];

% trang thai truoc
xkf_prev = [w_m_val; th_m_val; Tm_p_val];
xkf_prev = reshape(xkf_prev, 3, 1);

Pkf_prev = reshape(P_prev, 3, 3);

Q_kf = diag([q_w, q_th, q_tm]);
R_kf = diag([r_w, r_th]);

% du doan
x_pred = A_kf*xkf_prev + B_kf*Te_p_val;
P_pred = A_kf*Pkf_prev*A_kf.' + Q_kf;

% gain KF
S_kf   = C_kf*P_pred*C_kf.' + R_kf;
K_kf   = P_pred*C_kf' / S_kf;

% do luong
y_meas = [w_m_val; th_m_val];
y_meas = reshape(y_meas, 2, 1);

% cap nhat
x_hat  = x_pred + K_kf*(y_meas - C_kf*x_pred);
P_hat  = (eye(3) - K_kf*C_kf)*P_pred;

% tai uoc luong
Tm_hat = x_hat(3); % [Nm]

%% =========================================
% 4) TAO THAM CHIEU
% =========================================
t_now = clk_now_val; % [s]

[w_ref_rads_now, theta_ref_rad_now] = ref_at_time( ...
    mode_traj, t_now, Ts, ...
    alpha_max, omega_max, theta_max, ...
    omega_sin, wAref, t_step, ...
    t1_trap, t2_trap);

w_ref_rads_now = min(max(w_ref_rads_now, -OMEGA_MAX), OMEGA_MAX);
w_ref_rpm      = w_ref_rads_now * 60 / (2*pi); % [rpm]
theta_ref_rad  = theta_ref_rad_now; % [rad]

% vector tham chieu
Rs = zeros(2*Np,1);
for i = 1:Np
    ti = t_now + i*Ts;

    [wref_i, thref_i] = ref_at_time( ...
        mode_traj, ti, Ts, ...
        alpha_max, omega_max, theta_max, ...
        omega_sin, wAref, t_step, ...
        t1_trap, t2_trap);

    wref_i = min(max(wref_i, -OMEGA_MAX), OMEGA_MAX);

    Rs(2*i-1) = wref_i; % [rad/s]
    Rs(2*i)   = thref_i; % [rad]
end

%% ======================================================
% 5) MO HINH MPC
% ======================================================
A_mech = [1 - Ts*B/J, 0;
          Ts,         1];

B_mech = [Ts/J; 0];

% input mo hinh
u_prev = Te_p_val - Tm_hat; % [Nm]

% trang thai mo rong
A_aug  = [A_mech, B_mech;
          0,      0,      1];

B_aug  = [Ts/J;
          0;
          1];

C_aug  = [1 0 0;
          0 1 0];

% trang thai ban dau
x0 = [x_hat(1); x_hat(2); u_prev];
x0 = reshape(x0, 3, 1);

% xay dung F, G
F = zeros(2*Np, 3);
G = zeros(2*Np, Nc);

Apow_F = A_aug;
h = zeros(2, Np);
Apow_h = eye(3);

for i = 1:Np
    F(2*i-1:2*i, :) = C_aug * Apow_F;
    Apow_F = Apow_F * A_aug;

    h(:, i) = C_aug * Apow_h * B_aug;
    Apow_h = Apow_h * A_aug;
end

for j = 1:Nc
    for i = j:Np
        G(2*i-1:2*i, j) = h(:, i-j+1);
    end
end

%% =====================================
% 6) HAM MUC TIEU
% =====================================
Qy = zeros(2*Np, 2*Np);
for i = 1:Np
    Qy(2*i-1, 2*i-1) = Qw;
    Qy(2*i,   2*i  ) = Qth;
end

RuI = Ru * eye(Nc);

H = (G.' * Qy * G) + RuI;
f = (G.' * Qy * (F*x0 - Rs));

% rang buoc moment
Te_p_val_clip = max(-Te_max, min(Te_p_val, Te_max)); % [Nm]

S = tril(ones(Nc, Nc));

Mineq = [ S;
         -S];

Nineq = [ Te_max*ones(Nc,1) - Te_p_val_clip;
          Te_max*ones(Nc,1) + Te_p_val_clip ];

%% =====================================
% 7) GIAI QP HILDRETH
% =====================================
lambda = lambda_prev(:); % [-]
Te_next_val = Te_p_val_clip; % [Nm]

if new_tick
    H_reg = H + 1e-9*eye(Nc);

    H_inv_MineqT = H_reg \ (Mineq.');
    H_inv_f      = H_reg \ f;

    W     = Mineq * H_inv_MineqT;
    kvec  = Nineq + Mineq * H_inv_f;
    mcon  = size(Mineq, 1);

    for it = 1:max_iter
        lambda_old = lambda;
        for ii = 1:mcon
            sumi = W(ii,:)*lambda - W(ii,ii)*lambda(ii);
            wi   = (-kvec(ii) - sumi)/W(ii,ii);
            lambda(ii) = max(0, wi);
        end

        if (lambda - lambda_old).' * (lambda - lambda_old) < tol
            break;
        end
    end

    deltaU = -(H_reg \ (f + Mineq.'*lambda)); % [-]

    u_next_val  = u_prev + deltaU(1); % [Nm]

    Te_next_val = u_next_val + Tm_hat; % [Nm]
end

%% =====================================
% 8) XUAT KET QUA
% =====================================
Te_next_val = max(-Te_max, min(Te_next_val, Te_max)); % [Nm]

lambda_next = lambda; % [-]
Te_cmd      = Te_next_val; % [Nm]
Te_next     = Te_next_val; % [Nm]

% doi sang dong
iq_raw = (2/(3*p*pm)) * Te_cmd; % [A]
id_raw = 0.0; % [A]

iq_ref = max(-Iq_max, min(iq_raw, Iq_max)); % [A]
id_ref = max(-Iq_max, min(id_raw, Iq_max)); % [A]

xkf_next  = x_hat; % [-]
Pkf_next  = reshape(P_hat, 9, 1); % [-]

end

% ===========================
% Helper: Trajectory generator
% ===========================
function [wref, thref] = ref_at_time( ...
    mode_traj, t, Ts, ...
    alpha_max, omega_max, theta_max, ...
    omega_sin, wAref, t_step, ...
    t1_trap, t2_trap)

% OUTPUT:
% wref [rad/s] - toc do tham chieu
% thref [rad]  - goc tham chieu

switch mode_traj
    case 1 % Bell_shaped (S-curve)
        tc   = omega_max / alpha_max;
        jmax = alpha_max / tc;
        tm   = max(0, (theta_max - 2*jmax*tc^3)/omega_max);
        tf   = 4*tc + tm;
        kTs = t;

        if kTs < tc
            wref  = 0.5*jmax*(kTs)^2;
            thref = (1/6)*jmax*(kTs)^3;

        elseif kTs < 2*tc
            tau   = kTs - tc;
            wref  = 0.5*jmax*tc^2 + jmax*tc*tau - 0.5*jmax*tau^2;
            thref = (1/6)*jmax*tc^3 + 0.5*jmax*tc^2*tau + ...
                    0.5*jmax*tc*tau^2 - (1/6)*jmax*tau^3;

        elseif kTs < 2*tc + tm
            wref  = omega_max;
            thref = jmax*tc^3 + omega_max*(kTs - 2*tc);

        elseif kTs < 3*tc + tm
            tau   = kTs - 2*tc - tm;
            wref  = omega_max - 0.5*jmax*tau^2;
            thref = jmax*tc^3 + omega_max*tm + omega_max*tau - (1/6)*jmax*tau^3;

        elseif kTs < tf
            tau   = tf - kTs;
            wref  = 0.5*jmax*tau^2;
            thref = theta_max - (1/6)*jmax*tau^3;

        else
            wref = 0;
            thref = theta_max;
        end

    case 2 % Sin 
        % Bien do
        wAref = 300 * 2 * pi / 60; 
        
        % Chu ky dao dong 
        T_sin = 1.0;
        % Tan so goc omega = 2*pi / T
        omega_sin = 2 * pi / T_sin; 
        
        % Dung ham sin() cho van toc de dong co bat dau muot tu 0 rpm tai t=0. 
        % (Tranh dung cos() vi se gay nhay bac van toc len 300rpm ngay tu dau)
        wref  = wAref * sin(omega_sin * t);
        
        % Goc quay (tich phan chinh xac cua wref theo thoi gian)
        % Dam bao thref = 0 tai t = 0
        thref = (wAref / omega_sin) * (1 - cos(omega_sin * t));

    case 3 % Triangular trajectory (Quy dao tam giac)
        % 1. Thong so co ban cua tam giac
        T_period = 3.0; % Chu ky 3s
        A_rpm = 600.0;  % Bien do 300 rpm
        A_rad = A_rpm * 2 * pi / 60; % Chuyen sang rad/s
        
        % 2. Chia thoi gian trong 1 chu ky
        t_q = T_period / 4; % 0.75s (1/4 chu ky)
        
        % 3. Gia toc (do doc wref/t)
        alpha_tri = A_rad / t_q; 
        
        % 4. Dung mod() de quy dao lap lai vo han
        t_mod = mod(t, T_period);
        
        % 5. Tinh toan wref va thref tung giai doan
        if t_mod < t_q
            % Giai doan 1 (0 -> 0.75s): Tang tu 0 len +300 rpm
            wref  = alpha_tri * t_mod;
            thref = 0.5 * alpha_tri * t_mod^2;
            
        elseif t_mod < 3 * t_q
            % Giai doan 2 (0.75s -> 2.25s): Giam tu +300 rpm xuong -300 rpm
            tau = t_mod - t_q;
            % Goc tich luy duoc o cuoi Giai doan 1
            th_q = 0.5 * alpha_tri * t_q^2; 
            
            wref  = A_rad - alpha_tri * tau;
            thref = th_q + A_rad * tau - 0.5 * alpha_tri * tau^2;
            
        else
            % Giai doan 3 (2.25s -> 3.0s): Tang tu -300 rpm ve 0 rpm
            tau = t_mod - 3 * t_q;
            % Goc tich luy duoc o cuoi Giai doan 2 (ve mat toan hoc bang dung th_q)
            th_3q = 0.5 * alpha_tri * t_q^2; 
            
            wref  = -A_rad + alpha_tri * tau;
            thref = th_3q - A_rad * tau + 0.5 * alpha_tri * tau^2;
        end

    case 4 % Step
        % =========================================================
        % 1. CAI DAT THOI GIAN (TUY CHINH)
        % =========================================================
        t_step1 = 0.05; % Thoi diem bat dau chay GD 1
        t_step2 = 1.0;  % Thoi diem chuyen sang GD 2
        t_step3 = 1.5;  % Thoi diem chuyen sang GD 3
        t_step4 = 2.0;  % Thoi diem chuyen sang GD 4
        
        % T_trans: Thoi gian chuyen doi (giay).
        T_trans = 0.15; 
        
        % =========================================================
        % 2. CAI DAT TOC DO (SETPOINTS) -
        % =========================================================
        sp0 = 0;   % Toc do ban dau (truoc t_step1)
        sp1 = 300; % Toc do giai doan 1 (t_step1 -> t_step2)
        sp2 = 100; % Toc do giai doan 2 (t_step2 -> t_step3)
        sp3 = 200; % Toc do giai doan 3 (t_step3 -> t_step4)
        sp4 = 0;   % Toc do giai doan 4 (sau t_step4)
        
        % Doi toc do tu rpm sang rad/s (Tu dong)
        w_rad_0 = sp0 * 2 * pi / 60; 
        w_rad_1 = sp1 * 2 * pi / 60; 
        w_rad_2 = sp2 * 2 * pi / 60; 
        w_rad_3 = sp3 * 2 * pi / 60; 
        w_rad_4 = sp4 * 2 * pi / 60; 
        
        % --- TINH TOAN CAC GOC TICH LUY TAI CAC DIEM MOC ---
        th_start = w_rad_0 * t_step1; % Goc quay duoc truoc khi luon lan dau
        
        % Giai doan 1: sp0 -> sp1
        th_end_trans1 = th_start + (w_rad_0 + w_rad_1) * T_trans / 2; 
        th_end_hold1  = th_end_trans1 + w_rad_1 * (t_step2 - (t_step1 + T_trans));
        
        % Giai doan 2: sp1 -> sp2
        th_end_trans2 = th_end_hold1 + (w_rad_1 + w_rad_2) * T_trans / 2;
        th_end_hold2  = th_end_trans2 + w_rad_2 * (t_step3 - (t_step2 + T_trans));
        
        % Giai doan 3: sp2 -> sp3
        th_end_trans3 = th_end_hold2 + (w_rad_2 + w_rad_3) * T_trans / 2;
        th_end_hold3  = th_end_trans3 + w_rad_3 * (t_step4 - (t_step3 + T_trans));
        
        % Giai doan 4: sp3 -> sp4
        th_end_trans4 = th_end_hold3 + (w_rad_3 + w_rad_4) * T_trans / 2;

        % --- PHAN NHANH THOI GIAN DE XUAT RA wref, thref ---
        if t < t_step1
            % [1] Giai doan tinh dau tien
            wref  = w_rad_0;
            thref = w_rad_0 * t;
            
        elseif t < t_step1 + T_trans
            % [2] Luon tu sp0 len sp1
            tau = t - t_step1;
            ratio = tau / T_trans;
            delta_w = w_rad_1 - w_rad_0;
            
            wref  = w_rad_0 + delta_w * (3*ratio^2 - 2*ratio^3);
            thref = th_start + w_rad_0 * tau + delta_w * T_trans * (ratio^3 - 0.5*ratio^4);
            
        elseif t < t_step2
            % [3] Giu toc do sp1
            tau = t - (t_step1 + T_trans);
            wref  = w_rad_1;
            thref = th_end_trans1 + w_rad_1 * tau;
            
        elseif t < t_step2 + T_trans
            % [4] Luon tu sp1 sang sp2
            tau = t - t_step2;
            ratio = tau / T_trans;
            delta_w = w_rad_2 - w_rad_1;
            
            wref  = w_rad_1 + delta_w * (3*ratio^2 - 2*ratio^3);
            thref = th_end_hold1 + w_rad_1 * tau + delta_w * T_trans * (ratio^3 - 0.5*ratio^4);
            
        elseif t < t_step3
            % [5] Giu toc do sp2
            tau = t - (t_step2 + T_trans);
            wref  = w_rad_2;
            thref = th_end_trans2 + w_rad_2 * tau;
            
        elseif t < t_step3 + T_trans
            % [6] Luon tu sp2 sang sp3
            tau = t - t_step3;
            ratio = tau / T_trans;
            delta_w = w_rad_3 - w_rad_2;
            
            wref  = w_rad_2 + delta_w * (3*ratio^2 - 2*ratio^3);
            thref = th_end_hold2 + w_rad_2 * tau + delta_w * T_trans * (ratio^3 - 0.5*ratio^4);
            
        elseif t < t_step4
            % [7] Giu toc do sp3
            tau = t - (t_step3 + T_trans);
            wref  = w_rad_3;
            thref = th_end_trans3 + w_rad_3 * tau;
            
        elseif t < t_step4 + T_trans
            % [8] Luon tu sp3 sang sp4
            tau = t - t_step4;
            ratio = tau / T_trans;
            delta_w = w_rad_4 - w_rad_3;
            
            wref  = w_rad_3 + delta_w * (3*ratio^2 - 2*ratio^3);
            thref = th_end_hold3 + w_rad_3 * tau + delta_w * T_trans * (ratio^3 - 0.5*ratio^4);
            
        else
            % [9] Giu toc do cuoi sp4
            tau = t - (t_step4 + T_trans);
            wref  = w_rad_4;
            thref = th_end_trans4 + w_rad_4 * tau;
        end

    otherwise
        wref = 0;
        thref = 0;
end
end

== matlab function ClosedLoopPMSM_ASMO_MPC/SVPWM/SVPWM_main/XYZ Calculate ==
  settings: fimath=|
      | fimath(...
      | 'RoundMode', 'floor',...
      | 'OverflowMode', 'wrap',...
      | 'ProductMode', 'KeepLSB', 'ProductWordLength', 32,...
      | 'SumMode', 'KeepLSB', 'SumWordLength', 32,...
      | 'CastBeforeSum', false)
  data: Ualpha input; XYZ output; Ubeta input; Udc input; Ts input
function XYZ = XYZ_calc(Ualpha, Ubeta, Udc, Ts)

k1 = sqrt(3) * Ubeta;
k2 = (sqrt(3)/2) * Ubeta;
k3 = 3/2 * Ualpha;

k = Ts / Udc;

X = k * (k1);
Y = k * (k2 + k3);
Z = k * (k2 - k3);

XYZ = [X, Y, Z];
end

== matlab function ClosedLoopPMSM_ASMO_MPC/MATLAB Function1 ==
  data: sp input; w_in output; w_raw input; w_hat input; theta_e_raw input; theta_e_hat input; theta_in output; w_enc output; theta_e_enc output
function [w_in, theta_in, w_enc, theta_e_enc] = Synchronization(sp, w_raw, w_hat, theta_e_raw, theta_e_hat)
    % Chuyen mach trang thai (Encoder -> Sensorless) ket hop Dong bo hoa

    w_threshold = 0.0; 
    % Lay tri tuyet doi cua van toc dat
    abs_sp = abs(sp);

    if abs_sp < w_threshold
        % -------------------------------------------------------------
        % GIAI DOAN 1: TOC DO THAP 
        % -------------------------------------------------------------
        % Dung hoan toan tin hieu tu Encoder de dieu khien FOC
        w_in = w_raw;
        theta_in = theta_e_raw;
       
        w_enc = w_raw;
        theta_e_enc = theta_e_raw;
        
    else
        % -------------------------------------------------------------
        % GIAI DOAN 2: TOC DO CAO 
        % -------------------------------------------------------------
        % Chuyen sang dung hoan toan tin hieu tu Sensorless (ASMO)
        w_in = w_hat;
        theta_in = theta_e_hat;
       
        w_enc = w_hat;
        theta_e_enc = theta_e_hat;
    end
end
